simulink model "Cau7b"  (R2021b)
settings: Solver=VariableStepAuto  StartTime=0.0  StopTime=inf  RelTol=1e-3
libraries: commsink2 x2, commutil2 x2, commdigbbndam3 x2, commchan3 x1, commrandsrc3 x1
settings Model: Creator=ICTLAB  LastModifiedBy=ICTLAB
settings DataIOCC: ReturnWorkspaceOutputs=off

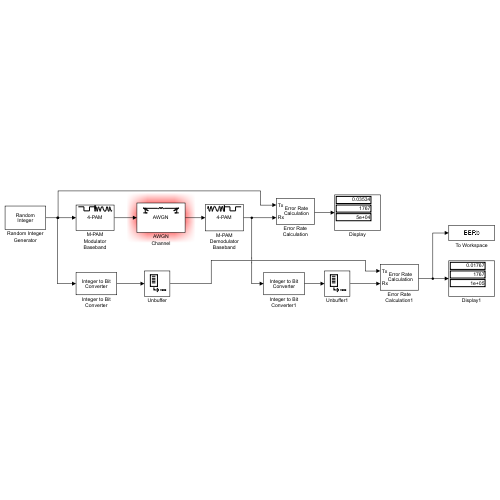
[thumbnail: Simulink's stored preview of the top-level diagram]
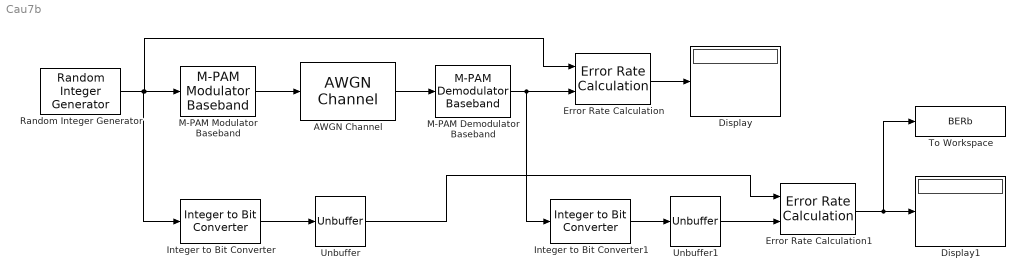
== system Cau7b ==
  AWGN Channel : commchan3/AWGN Channel  InputProcessing=Columns as channels (frame based)  seed=67  noiseMode="Signal to noise ratio  (Eb/No)"  EbNodB=EbNo  EsNodB=10  SNRdB=10  bitsPerSym=2  Ps=5  Tsym=1/4000  variance=1
  Display : Display
  Display1 : Display
  Error Rate Calculation : commsink2/Error Rate Calculation  N=0  st_delay=0  cp_mode=Entire frame  subframe=[]  PMode=Port  WsName=ErrorVec  RsMode2=off  stop=off  numErr=100  maxBits=1e6
  Error Rate Calculation1 : commsink2/Error Rate Calculation  N=0  st_delay=0  cp_mode=Entire frame  subframe=[]  PMode=Port  WsName=ErrorVec  RsMode2=off  stop=on  numErr=1e4  maxBits=1e5
  Integer to Bit Converter : commutil2/Integer to Bit Converter  nbits=2  signedInputValues=Unsigned  bitOrder=MSB first  outDtype=Inherit via internal rule
  Integer to Bit Converter1 : commutil2/Integer to Bit Converter  nbits=2  signedInputValues=Unsigned  bitOrder=MSB first  outDtype=Inherit via internal rule
  M-PAM Demodulator Baseband : commdigbbndam3/M-PAM Demodulator Baseband  M=4  OutType=Integer  Dec=Gray  PowType=Min. distance between symbols  MinDist=2  AvgPow=1  PeakPow=1  outDtype1=Inherit via internal rule  outDtype2=Inherit via internal rule  denormFactorWordLen=16  denormFactorDataTypeStr=Inherit: Same word length as input  denormFactorLastDataTypeStr=Inherit: Same word length as input  prodOutWordLen=16  prodOutRoundingMode=Floor  prodOutOverflowMode=Wrap  prodOutOvFlMode=off  prodOutOvFlModeLastStrValue=off  sumWordLen=16
      settings: SourceProductBaseCode=CM
  M-PAM Modulator Baseband : commdigbbndam3/M-PAM Modulator Baseband  M=4  InType=Integer  Enc=Gray  PowType=Min. distance between symbols  MinDist=2  AvgPow=1  PeakPow=1  outDtype=double  outWordLen=16  outUDDataType=sfix(16)  outFracLenMode=Best precision  outFracLen=15  outDataTypeStr=double  outLastDataTypeStr=double
      settings: SourceProductBaseCode=CM
  Random Integer Generator : commrandsrc3/Random Integer Generator  SetSize=4  SeedSource=Auto  Seed=0  SampleTime=1/4000  SamplesPerFrame=1  OutputDataType=double  SimulateUsing=Interpreted execution
  To Workspace : ToWorkspace  VariableName=BERb  SampleTime=-1
      settings: MaxDataPoints=1
  Unbuffer : Unbuffer
  Unbuffer1 : Unbuffer
  wires:
  Random Integer Generator/1 -> Integer to Bit Converter/1, Error Rate Calculation/1, M-PAM Modulator Baseband/1
  M-PAM Modulator Baseband/1 -> AWGN Channel/1
  AWGN Channel/1 -> M-PAM Demodulator Baseband/1
  M-PAM Demodulator Baseband/1 -> Integer to Bit Converter1/1, Error Rate Calculation/2
  Error Rate Calculation/1 -> Display/1
  Integer to Bit Converter/1 -> Unbuffer/1
  Integer to Bit Converter1/1 -> Unbuffer1/1
  Unbuffer1/1 -> Error Rate Calculation1/2
  Unbuffer/1 -> Error Rate Calculation1/1
  Error Rate Calculation1/1 -> To Workspace/1, Display1/1
